simulink model "PlantModel_NN"  (R2018b)
settings: Solver=VariableStepAuto  StartTime=0.0  StopTime=10.0  RelTol=1e-3
values from neighbouring files (symbols this model uses):
  A = 1e-6    (= 1e-06)    [IC_4DOF_new.m]    (also in IC_4DOF_new2.m; ODE_4DOF_new.m = [zeros(4), eye(4); C+Hs, omega_dim*G+Hd/omega_dim]; ODE_MAGLEV_4DOF.m = [zeros(4), eye(4); C+Hs, (omega_dim*G)+(Hd/omega_dim)]; PID_Test2_.m = [zeros(4), eye(4); C+Hs, (omega_dim*G)+(Hd/omega_dim)])
  a1_dim = a1/Sl    (= 0.409090909091)    [IC_4DOF_new.m]    (also in IC_4DOF_new2.m; PID_Test2_.m; var_IC_4DOF.m)
  a2_dim = a2/Sl    (= 0.409090909091)    [IC_4DOF_new.m]    (also in IC_4DOF_new2.m; PID_Test2_.m; var_IC_4DOF.m)
  alpha1 = alpha1/Sbeta    (= 0)    [IC_4DOF_new.m]    (also in IC_4DOF_new2.m = 2.2; PID_Test2_.m; var_IC_4DOF.m)
  Ax_dim = Ax/Sf    (= 0.000833333333333)    [IC_4DOF_new.m]    (also in IC_4DOF_new2.m; PID_Test2_.m; var_IC_4DOF.m)
  beta1 = beta1/Sbeta    (= 0)    [IC_4DOF_new.m]    (also in IC_4DOF_new2.m = 1.65; PID_Test2_.m; var_IC_4DOF.m)
  C_ss = [Ident zer]    [PID_Test2_.m]
  D_ss = zer    [PID_Test2_.m]
  delta_dim = delta_dim/Sx    (= 1)    [IC_4DOF_new.m]    (also in IC_4DOF_new2.m; PID_Test2_.m; var_IC_4DOF.m)
  i0_dim = i0/Si    (= 0)    [IC_4DOF_new.m]    (also in IC_4DOF_new2.m = 0.05; PID_Test2_.m = 0.0007; var_IC_4DOF.m = 0.5)
  omega_dim = omega/Sw    [IC_4DOF_new.m]    (also in IC_4DOF_new2.m; ODE_4DOF_new.m = par(11); ODE_MAGLEV_4DOF.m = par(11); PID_Test2_.m)
  P2 = par(22)    [Force_4DOF.m]    (also in IC_4DOF_new.m = 2.178; IC_4DOF_new2.m = 2.178; PID_Test2_.m = 8.714; var_IC_4DOF.m = 2.178)
  p_dim = nu*2*pi/Sw    [AFC_4DOF_NM.m]    (also in IC_4DOF_new.m = p/Sw; IC_4DOF_new2.m = p/Sw; PID_Test2_.m = p/Sw; var_IC_4DOF.m = p/Sw)
  Pk = par(15)    [Force_4DOF.m]    (also in IC_4DOF_new.m = 8.41666666667e-05; IC_4DOF_new2.m = ka*P_e/(cm*R_e*delta_dim^3); PID_Test2_.m = 1000000; var_IC_4DOF.m = ka*P_e/(cm*R_e*delta_dim^3))
  Px_dim = Px/Sf    (= 0)    [IC_4DOF_new.m]    (also in IC_4DOF_new2.m = 1.62337662338; PID_Test2_.m; var_IC_4DOF.m)
  Py_dim = Py/Sf    (= 0)    [IC_4DOF_new.m]    (also in IC_4DOF_new2.m = 1.62337662338; PID_Test2_.m; var_IC_4DOF.m)
  x1 = x1/Sx    (= 0.5)    [IC_4DOF_new.m]    (also in IC_4DOF_new2.m; PID_Test2_.m; var_IC_4DOF.m)
  y1 = y1/Sx    (= 0.25)    [IC_4DOF_new.m]    (also in IC_4DOF_new2.m; PID_Test2_.m; var_IC_4DOF.m)
  zer_o = [0;0;0;0]    [PID_Test2_.m]
libraries: dspmtrx3 x2, cstblocks x1
settings Model: Creator=first  LastModifiedBy=first
settings DebuggingCC: UnderSpecifiedDimensionMsg=warning

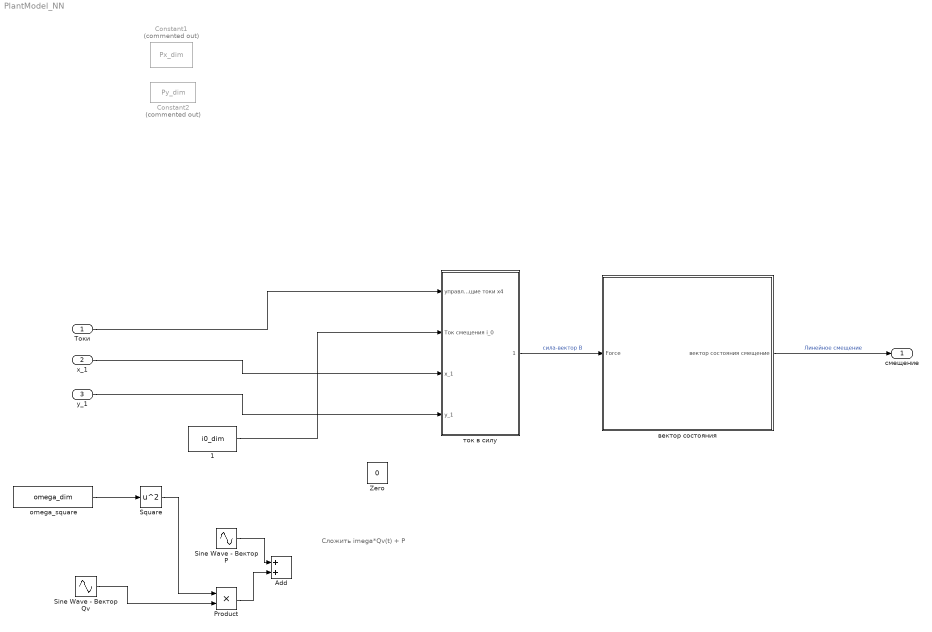
== system PlantModel_NN ==
  note: Сложить imega*Qv(t) + P
  Токи : Inport
  x_1 : Inport  Port=2
  y_1 : Inport  Port=3
  " 1" : Constant  Value=i0_dim
  " вектор состояния " : Subsystem
  Add : Sum
  Constant1 : Constant  Commented=on  Value=Px_dim
  Constant2 : Constant  Commented=on  Value=Py_dim
  Product : Product
  Sine Wave - Вектор P : Sin  Amplitude=Ax_dim  Bias=Px_dim  Frequency=p_dim  SampleTime=1
  Sine Wave - Вектор Qv : Sin  Amplitude=Ax_dim  Bias=Px_dim  Frequency=p_dim  SampleTime=1
  Square : Math  Operator=square  SaturateOnIntegerOverflow=on
  Zero : Constant  Value=0  OutDataTypeStr=Inherit: Inherit via back propagation
  omega_square : Constant  Value=omega_dim
  "ток в силу " : Subsystem
  смещение : Outport
  wires:
  omega_square/1 -> Square/1
  Square/1 -> Product/1
  Product/1 -> Add/2
  Токи/1 -> "ток в силу "/1(управляющие токи x4)
  " вектор состояния "/1(вектор состояния смещение) -> смещение/1  "Линейное смещение"
  "ток в силу "/1(" ") -> " вектор состояния "/1(Force)  "сила-вектор B"
  Sine Wave - Вектор Qv/1 -> Product/2
  Sine Wave - Вектор P/1 -> Add/1
  x_1/1 -> "ток в силу "/3(x_1)
  y_1/1 -> "ток в силу "/4(y_1)
  " 1"/1 -> "ток в силу "/2(Ток смещения i_0)

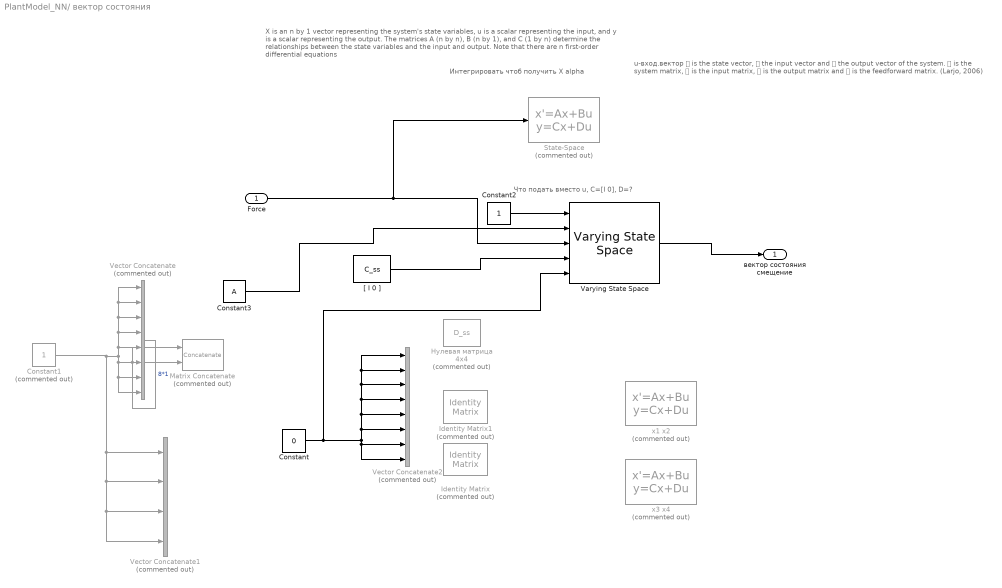
== system PlantModel_NN/ вектор состояния  ==
  note: Что подать вместо u, C=[I 0], D=?
  note: u-вход.вектор
      |  𝒙 is the state vector, 𝒖 the input vector and 𝒚 the output vector of the system.
      | 𝐀 is the system matrix, 𝐁 is the input matrix, 𝐂 is the output matrix and 𝐃 is the feedforward matrix.
      | (Larjo, 2006)
  note: X is an n by 1 vector representing the system's state variables, u is a scalar representing the input, and y is a scalar representing the output.
      |  The matrices A (n by n), B (n by 1), and C (1 by n) determine the relationships between the state variables and the input and output.
      | Note that there are n first-order differential equations
  note: Интегрировать чтоб получить X alpha
  Force : Inport
  Constant : Constant  Value=0
  Constant1 : Constant  Commented=on
  Constant2 : Constant
  Constant3 : Constant  Value=A
  Identity Matrix : dspmtrx3/Identity Matrix  Commented=on  Inherit=off  N=4  Ts=1  dataType=double  isSigned=on  wordLen=16  udDataType=sfix(16)  fracBitsMode=Best precision  numFracBits=15  OutDataTypeStr=double  LastOutDataTypeStr=double
      settings: SourceProductName=DSP System Toolbox
  Identity Matrix1 : dspmtrx3/Identity Matrix  Commented=on  Inherit=off  N=8  Ts=1  dataType=double  isSigned=on  wordLen=16  udDataType=sfix(16)  fracBitsMode=Best precision  numFracBits=15  OutDataTypeStr=double  LastOutDataTypeStr=double
      settings: SourceProductName=DSP System Toolbox
  Matrix Concatenate : Concatenate  Commented=on  Mode=Multidimensional array  ConcatenateDimension=8
  State-Space : StateSpace  Commented=on  InitialCondition=0
  Varying State Space : cstblocks/Linear Parameter Varying/Varying State Space  x0=0  xNames=''  OutputX=on  OutputDX=on
      settings: SourceProductName=Control System Toolbox
  Vector Concatenate : Concatenate  Commented=on  NumInputs=8
  Vector Concatenate1 : Concatenate  Commented=on  NumInputs=4
  Vector Concatenate2 : Concatenate  Commented=on  NumInputs=8
  "[ I 0 ] " : Constant  Value=C_ss
  x1 x2 : StateSpace  Commented=on  InitialCondition=0
  x3 x4 : StateSpace  Commented=on  InitialCondition=0
  Нулевая матрица 4x4 : Constant  Commented=on  Value=D_ss
  вектор состояния смещение : Outport
  wires:
  Force/1 -> Varying State Space/3, State-Space/1
  Constant3/1 -> Varying State Space/2
  Constant1/1 -> Vector Concatenate1/4, Vector Concatenate1/3, Vector Concatenate1/2, Vector Concatenate1/1, Vector Concatenate/4, Vector Concatenate/1, Vector Concatenate/2, Vector Concatenate/3, Vector Concatenate/5, Vector Concatenate/8, Vector Concatenate/7, Vector Concatenate/6
  Vector Concatenate/1 -> Matrix Concatenate/1, Matrix Concatenate/2  "8*1"
  Constant/1 -> Varying State Space/5, Vector Concatenate2/8, Vector Concatenate2/7, Vector Concatenate2/6, Vector Concatenate2/4, Vector Concatenate2/3, Vector Concatenate2/2, Vector Concatenate2/1, Vector Concatenate2/5
  Varying State Space/2 -> вектор состояния смещение/1
  "[ I 0 ] "/1 -> Varying State Space/4
  Constant2/1 -> Varying State Space/1

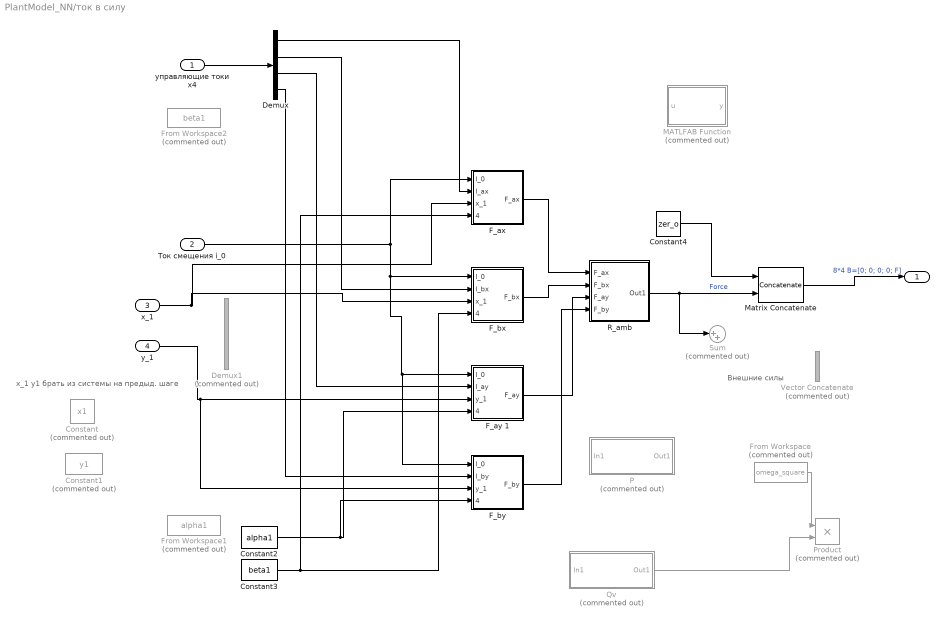
== system PlantModel_NN/ток в силу  ==
  note: Внешние силы
  note: x_1 y1 брать из системы на предыд. шаге
  управляющие токи x4 : Inport
  Ток смещения i_0 : Inport  Port=2
  x_1 : Inport  Port=3
  y_1 : Inport  Port=4
  Constant : Constant  Commented=on  Value=x1
  Constant1 : Constant  Commented=on  Value=y1
  Constant2 : Constant  Value=alpha1
  Constant3 : Constant  Value=beta1
  Constant4 : Constant  Value=zer_o
  Demux : Demux
  Demux1 : Demux  Commented=on
  F_ax : Subsystem
  F_ay 1 : Subsystem
  F_bx : Subsystem
  F_by : Subsystem
  From Workspace : FromWorkspace  Commented=on  VariableName=omega_square  SampleTime=0
  From Workspace1 : FromWorkspace  Commented=on  VariableName=alpha1  SampleTime=0
  From Workspace2 : FromWorkspace  Commented=on  VariableName=beta1  SampleTime=0
  MATLFAB Function : MATLAB Function  Commented=on  TreatAsAtomicUnit=on
  Matrix Concatenate : Concatenate  Mode=Multidimensional array
  P : Subsystem  Commented=on
  Product : Product  Commented=on
  Qv : Subsystem  Commented=on
  R_amb : Subsystem
  Sum : Sum  Commented=on  Inputs=|++
  Vector Concatenate : Concatenate  Commented=on
  " " : Outport
  wires:
  F_ax/1(F_ax) -> R_amb/1(F_ax)
  F_bx/1(F_bx) -> R_amb/2(F_bx)
  F_ay 1/1(F_ay) -> R_amb/3(F_ay)
  F_by/1(F_by) -> R_amb/4(F_by)
  From Workspace/1 -> Product/1
  Qv/1(Out1) -> Product/2
  Ток смещения i_0/1 -> F_by/1(I_0), F_ay 1/1(I_0), F_bx/1(I_0), F_ax/1(I_0)
  управляющие токи x4/1 -> Demux/1
  Demux/1 -> F_ax/2(I_ax)
  Demux/2 -> F_bx/2(I_bx)
  Demux/3 -> F_ay 1/2(I_ay)
  Demux/4 -> F_by/2(I_by)
  Constant2/1 -> F_by/4(alpha_1), F_ay 1/4(alpha_1)
  Constant3/1 -> F_bx/4(betta_1), F_ax/4(betta_1)
  Matrix Concatenate/1 -> " "/1  "8*4 B=[0; 0; 0; 0; F]"
  Constant4/1 -> Matrix Concatenate/1
  x_1/1 -> F_bx/3(x_1), F_ax/3(x_1)
  y_1/1 -> F_by/3(y_1), F_ay 1/3(y_1)
  R_amb/1(Out1) -> Matrix Concatenate/2, Sum/1  "Force"
  ? -> Sum/2

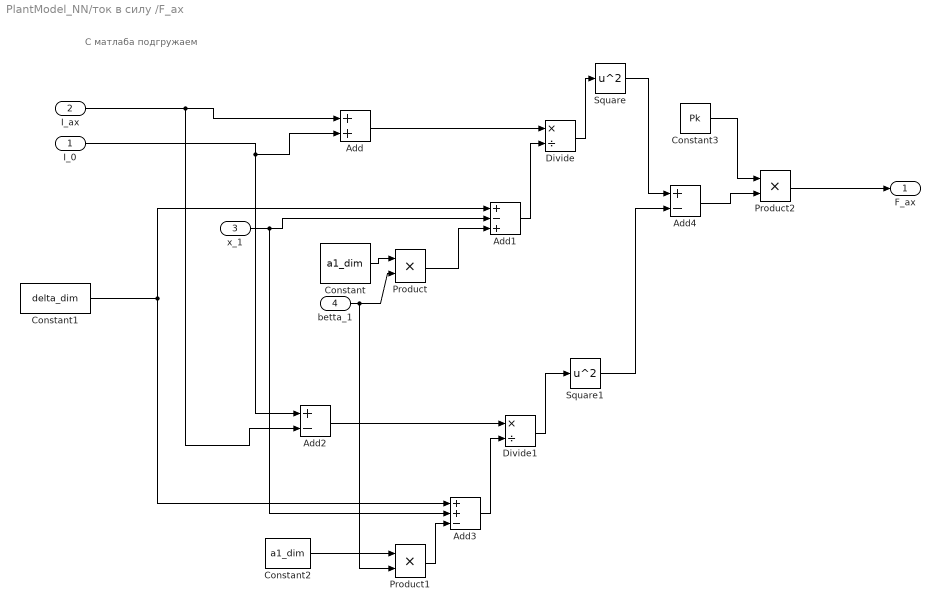
== system PlantModel_NN/ток в силу /F_ax ==
  note: С матлаба подгружаем
  I_0 : Inport
  I_ax : Inport  Port=2
  x_1 : Inport  Port=3
  betta_1 : Inport  Port=4
  Add : Sum
  Add1 : Sum  Inputs=+-+
  Add2 : Sum  Inputs=+-
  Add3 : Sum  Inputs=++-
  Add4 : Sum  Inputs=+-
  Constant : Constant  Value=a1_dim
  Constant1 : Constant  Value=delta_dim
  Constant2 : Constant  Value=a1_dim
  Constant3 : Constant  Value=Pk
  Divide : Product  Inputs=*/
  Divide1 : Product  Inputs=*/
  Product : Product
  Product1 : Product
  Product2 : Product
  Square : Math  Operator=square  SaturateOnIntegerOverflow=on
  Square1 : Math  Operator=square  SaturateOnIntegerOverflow=on
  F_ax : Outport
  wires:
  Product2/1 -> F_ax/1
  Constant/1 -> Product/1
  Product/1 -> Add1/3
  Add1/1 -> Divide/2
  Add/1 -> Divide/1
  Divide/1 -> Square/1
  Product1/1 -> Add3/3
  Add2/1 -> Divide1/1
  Constant2/1 -> Product1/1
  I_ax/1 -> Add2/2, Add/1
  Add3/1 -> Divide1/2
  x_1/1 -> Add1/2, Add3/2
  Divide1/1 -> Square1/1
  I_0/1 -> Add/2, Add2/1
  betta_1/1 -> Product/2, Product1/2
  Square/1 -> Add4/1
  Square1/1 -> Add4/2
  Constant3/1 -> Product2/1
  Add4/1 -> Product2/2
  Constant1/1 -> Add1/1, Add3/1

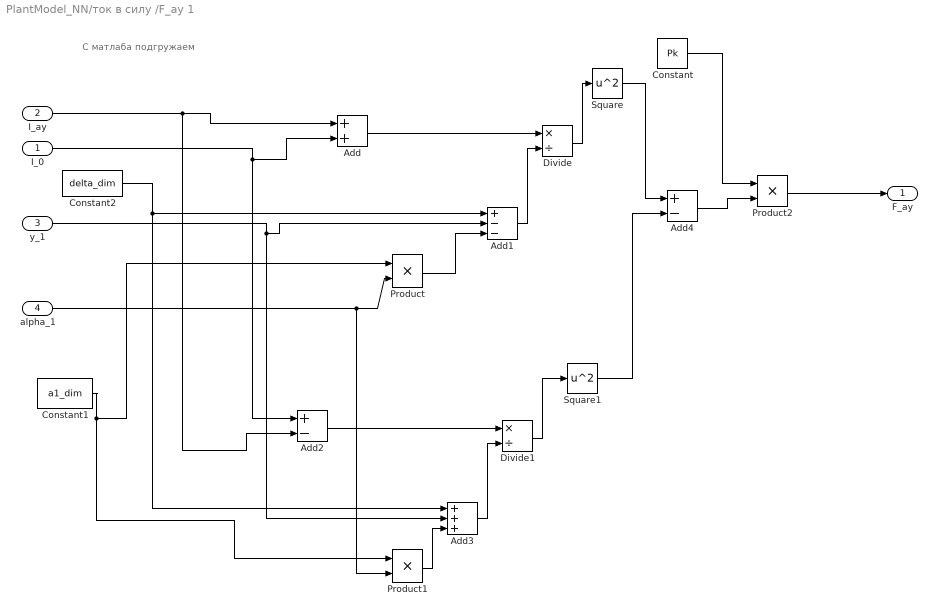
== system PlantModel_NN/ток в силу /F_ay 1 ==
  note: С матлаба подгружаем
  I_0 : Inport
  I_ay : Inport  Port=2
  y_1 : Inport  Port=3
  alpha_1 : Inport  Port=4
  Add : Sum
  Add1 : Sum  Inputs=+--
  Add2 : Sum  Inputs=+-
  Add3 : Sum  Inputs=+++
  Add4 : Sum  Inputs=+-
  Constant : Constant  Value=Pk
  Constant1 : Constant  Value=a1_dim
  Constant2 : Constant  Value=delta_dim
  Divide : Product  Inputs=*/
  Divide1 : Product  Inputs=*/
  Product : Product
  Product1 : Product
  Product2 : Product
  Square : Math  Operator=square  SaturateOnIntegerOverflow=on
  Square1 : Math  Operator=square  SaturateOnIntegerOverflow=on
  F_ay : Outport
  wires:
  Product2/1 -> F_ay/1
  Product/1 -> Add1/3
  Add1/1 -> Divide/2
  Add/1 -> Divide/1
  Divide/1 -> Square/1
  Product1/1 -> Add3/3
  Add2/1 -> Divide1/1
  Constant1/1 -> Product1/1, Product/1
  I_ay/1 -> Add2/2, Add/1
  Add3/1 -> Divide1/2
  y_1/1 -> Add1/2, Add3/2
  Divide1/1 -> Square1/1
  I_0/1 -> Add/2, Add2/1
  alpha_1/1 -> Product/2, Product1/2
  Square/1 -> Add4/1
  Square1/1 -> Add4/2
  Constant/1 -> Product2/1
  Add4/1 -> Product2/2
  Constant2/1 -> Add3/1, Add1/1

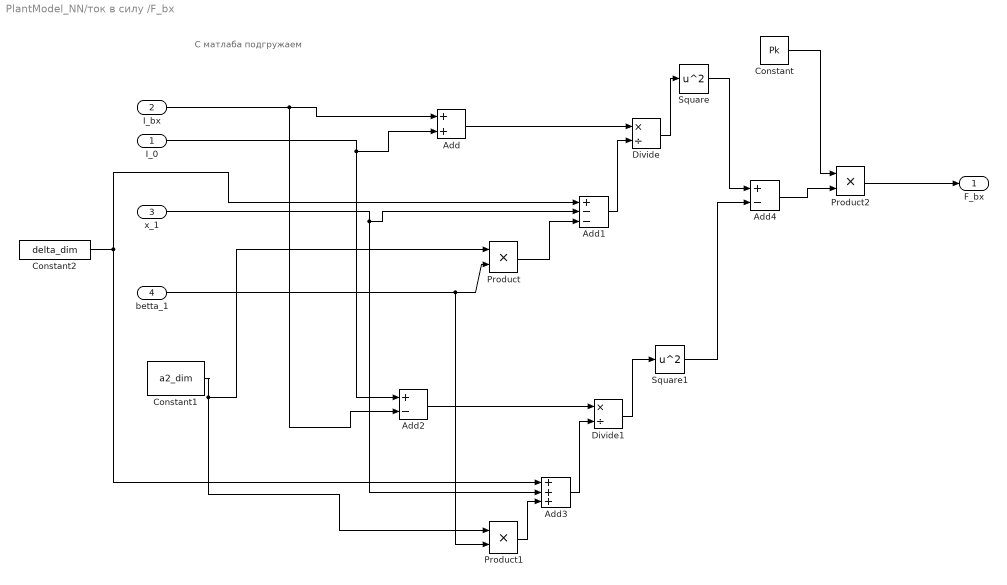
== system PlantModel_NN/ток в силу /F_bx ==
  note: С матлаба подгружаем
  I_0 : Inport
  I_bx : Inport  Port=2
  x_1 : Inport  Port=3
  betta_1 : Inport  Port=4
  Add : Sum
  Add1 : Sum  Inputs=+--
  Add2 : Sum  Inputs=+-
  Add3 : Sum  Inputs=+++
  Add4 : Sum  Inputs=+-
  Constant : Constant  Value=Pk
  Constant1 : Constant  Value=a2_dim
  Constant2 : Constant  Value=delta_dim
  Divide : Product  Inputs=*/
  Divide1 : Product  Inputs=*/
  Product : Product
  Product1 : Product
  Product2 : Product
  Square : Math  Operator=square  SaturateOnIntegerOverflow=on
  Square1 : Math  Operator=square  SaturateOnIntegerOverflow=on
  F_bx : Outport
  wires:
  Product2/1 -> F_bx/1
  Product/1 -> Add1/3
  Add1/1 -> Divide/2
  Add/1 -> Divide/1
  Divide/1 -> Square/1
  Product1/1 -> Add3/3
  Add2/1 -> Divide1/1
  Constant1/1 -> Product1/1, Product/1
  I_bx/1 -> Add2/2, Add/1
  Add3/1 -> Divide1/2
  x_1/1 -> Add1/2, Add3/2
  Divide1/1 -> Square1/1
  I_0/1 -> Add/2, Add2/1
  betta_1/1 -> Product/2, Product1/2
  Square/1 -> Add4/1
  Square1/1 -> Add4/2
  Constant/1 -> Product2/1
  Add4/1 -> Product2/2
  Constant2/1 -> Add1/1, Add3/1

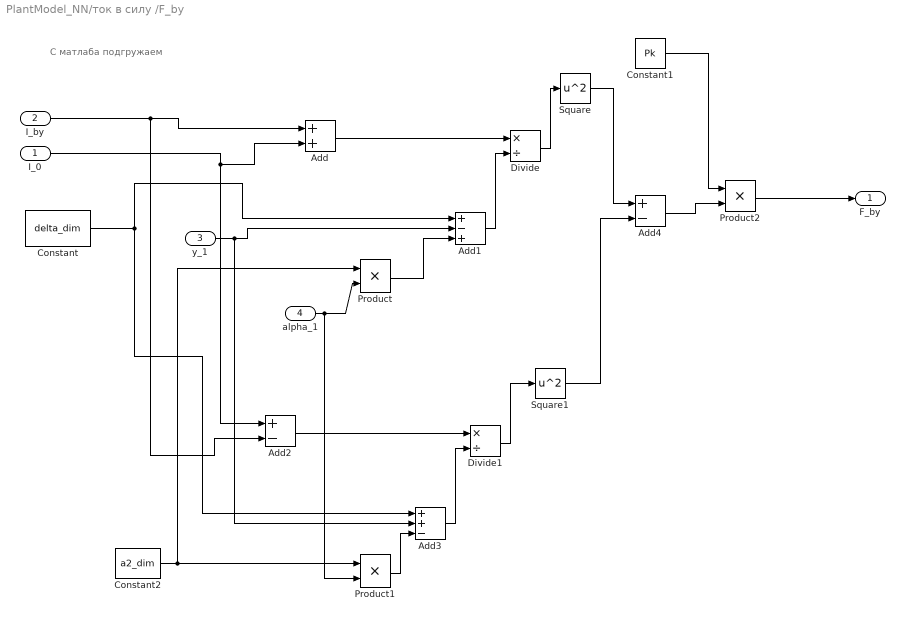
== system PlantModel_NN/ток в силу /F_by ==
  note: С матлаба подгружаем
  I_0 : Inport
  I_by : Inport  Port=2
  y_1 : Inport  Port=3
  alpha_1 : Inport  Port=4
  Add : Sum
  Add1 : Sum  Inputs=+-+
  Add2 : Sum  Inputs=+-
  Add3 : Sum  Inputs=++-
  Add4 : Sum  Inputs=+-
  Constant : Constant  Value=delta_dim
  Constant1 : Constant  Value=Pk
  Constant2 : Constant  Value=a2_dim
  Divide : Product  Inputs=*/
  Divide1 : Product  Inputs=*/
  Product : Product
  Product1 : Product
  Product2 : Product
  Square : Math  Operator=square  SaturateOnIntegerOverflow=on
  Square1 : Math  Operator=square  SaturateOnIntegerOverflow=on
  F_by : Outport
  wires:
  Product2/1 -> F_by/1
  Constant2/1 -> Product/1, Product1/1
  Product/1 -> Add1/3
  Add1/1 -> Divide/2
  Add/1 -> Divide/1
  Divide/1 -> Square/1
  Product1/1 -> Add3/3
  Add2/1 -> Divide1/1
  I_by/1 -> Add2/2, Add/1
  Add3/1 -> Divide1/2
  y_1/1 -> Add1/2, Add3/2
  Constant/1 -> Add1/1, Add3/1
  Divide1/1 -> Square1/1
  I_0/1 -> Add/2, Add2/1
  alpha_1/1 -> Product/2, Product1/2
  Square/1 -> Add4/1
  Square1/1 -> Add4/2
  Constant1/1 -> Product2/1
  Add4/1 -> Product2/2

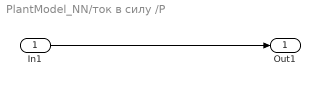
== system PlantModel_NN/ток в силу /P ==
  In1 : Inport
  Out1 : Outport
  wires:
  In1/1 -> Out1/1

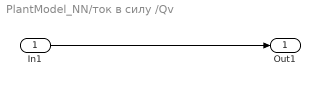
== system PlantModel_NN/ток в силу /Qv ==
  In1 : Inport
  Out1 : Outport
  wires:
  In1/1 -> Out1/1

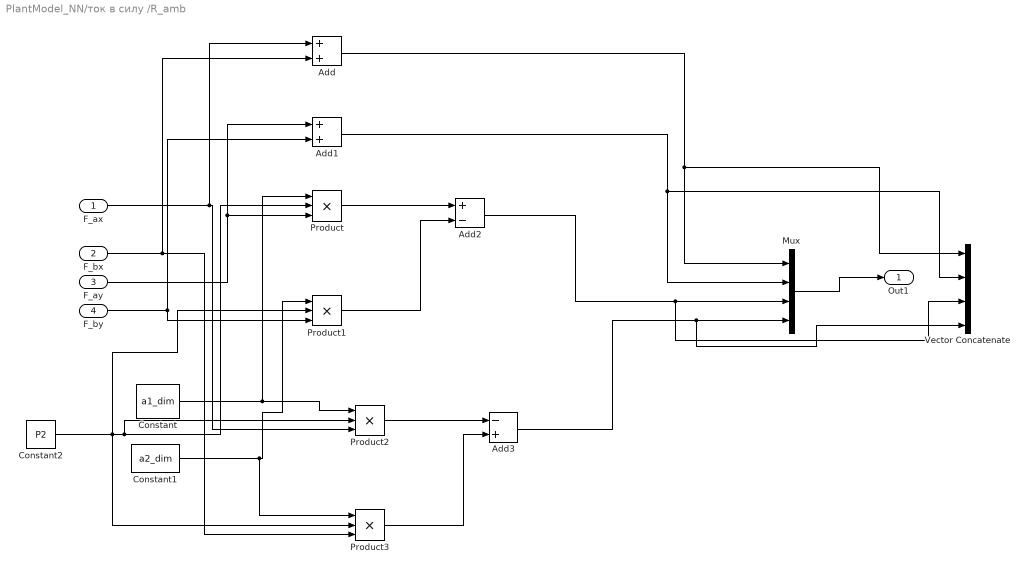
== system PlantModel_NN/ток в силу /R_amb ==
  F_ax : Inport
  F_bx : Inport  Port=2
  F_ay : Inport  Port=3
  F_by : Inport  Port=4
  Add : Sum
  Add1 : Sum
  Add2 : Sum  Inputs=+-
  Add3 : Sum  Inputs=-+
  Constant : Constant  Value=a1_dim
  Constant1 : Constant  Value=a2_dim
  Constant2 : Constant  Value=P2
  Mux : Mux
  Product{,1..3} (4 alike) : Product  Inputs=3
  Vector Concatenate : Concatenate  NumInputs=4
  Out1 : Outport  PortDimensions=4
  wires:
  F_ax/1 -> Product2/3, Add/1
  F_bx/1 -> Product3/3, Add/2
  Add/1 -> Mux/1, Vector Concatenate/1
  F_ay/1 -> Product/3, Add1/1
  F_by/1 -> Product1/3, Add1/2
  Add1/1 -> Mux/2, Vector Concatenate/2
  Constant/1 -> Product2/1, Product/1
  Product/1 -> Add2/1
  Constant1/1 -> Product3/1, Product1/1
  Product1/1 -> Add2/2
  Add2/1 -> Vector Concatenate/3, Mux/3
  Product3/1 -> Add3/2
  Product2/1 -> Add3/1
  Add3/1 -> Vector Concatenate/4, Mux/4
  Constant2/1 -> Product/2, Product2/2, Product3/2, Product1/2
  Mux/1 -> Out1/1

== matlab function PlantModel_NN/ток в силу /MATLFAB Function ==
  data: u input; y output
function y = fcn(u)

y = u;
